simulink model "test_xh2fl"  (R2016a)
settings: Solver=VariableStepAuto  StartTime=0.0  StopTime=1e3  RelTol=1e-3
libraries: simCryogenics_lib x7, nesl_utility x1
settings Model: Creator=FB229602  LastModifiedBy=FB229602
settings GRTTargetCC: GeneratePreprocessorConditionals=Use local settings
settings SimscapeCC: SimscapeLogType=all  SimscapeLogLimitData=off

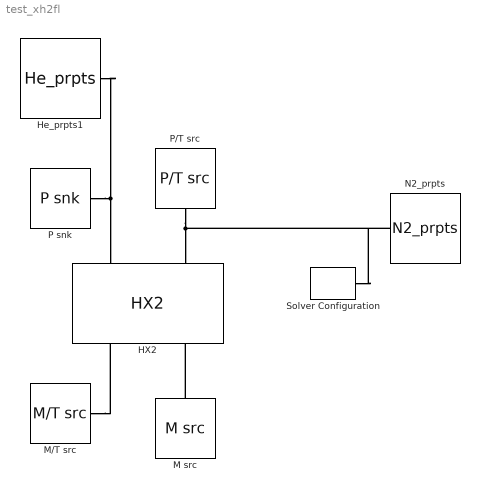
== system test_xh2fl ==
  HX2 : simCryogenics_lib/Elements/HX2  N=9  Vh=2.3e-3 m^3  Vc=2.3e-3 m^3  M=13 kg  Kh=0 s*bar/kg  Kc=0 s*bar/kg  h=48 J/s/K  Th0=300 K  Ph0=16 bar  Mh0=0.01*5 kg/s  Tc0=200 K  Pc0=1 bar  Mc0=0.01 kg/s
  He_prpts1 : simCryogenics_lib/Utilities/He_prpts  P_min=0.5 bar  P_max=20 bar  T_min=150 K  T_max=350 K  N=100  Mol=4.0026 * (10 ^ (- 3)) kg/mol
  M src : simCryogenics_lib/Sources_Sinks/M src  M=0.01*5 kg/s
  M/T src : simCryogenics_lib/Sources_Sinks/M//T src  M=0.01 kg/s  T=200 K
  N2_prpts : simCryogenics_lib/Utilities/N2_prpts  P_min=0.5 bar  T_min=70 K  T_max=320 K  P_max=20 bar  Mol=4.0026 * (10 ^ (- 3)) kg/mol
  P snk : simCryogenics_lib/Sources_Sinks/P snk  P=1 bar
  P/T src : simCryogenics_lib/Sources_Sinks/P//T src  P=16 bar  T=300 K
  Solver Configuration : nesl_utility/Solver Configuration  PhysicalDomain=network_engine_domain  SubClassName=solver  LeftPortType=input  RightPortType=generic  Accelerate=off  Tones=[]  Harmonics=[]  SimulateNoise=off  Profile=off  UseLocalSampling=off  EnableSwitchedLinearOptims=on  FrequencyDomain=off  UseCCode=off  RelTol=0.001  AbsTol=1e-06  MinStep=1e-09  ToWorkspace=off  RevertToSquareIcSolve=off  NumHomotopyIterations=100  PhasorMode=off  PhasorModeNumHarmonics=1  OverrideAbsTol=off  DoDC=off  ResidualTolerance=1e-09  UseLocalSolver=off  LocalSolverChoice=NE_BACKWARD_EULER_ADVANCER  LocalSolverSampleTime=0.001  DoFixedCost=off  MaxNonlinIter=3  MaxModeIter=2  LinearAlgebra=Sparse  DelaysMemoryBudget=1024  AutomaticFiltering=on  FilteringTimeConstant=0.001
  connections:
  P/T src/RConn1 -- Solver Configuration/RConn1 -- N2_prpts/RConn1 -- HX2/LConn2
  M src/RConn1 -- HX2/RConn2
  P snk/RConn1 -- HX2/LConn1 -- He_prpts1/RConn1
  M/T src/RConn1 -- HX2/RConn1
